simulink model "Sensor_Process"  (R2025b)
settings: Solver=VariableStepAuto  StartTime=0.0  StopTime=10.0  RelTol=1e-3
values from neighbouring files (symbols this model uses):
  sensor_distance_table = [100 80 60 40 20 5]    [run_MAIN.m]
  sensor_voltage_breakpoints = [0 1 2 3 4 5]    [run_MAIN.m]
settings Model: Creator=Mohamed  LastModifiedBy=Mohamed

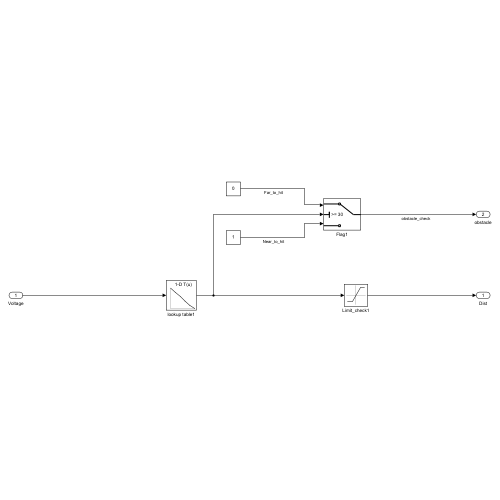
[thumbnail: Simulink's stored preview of the top-level diagram]
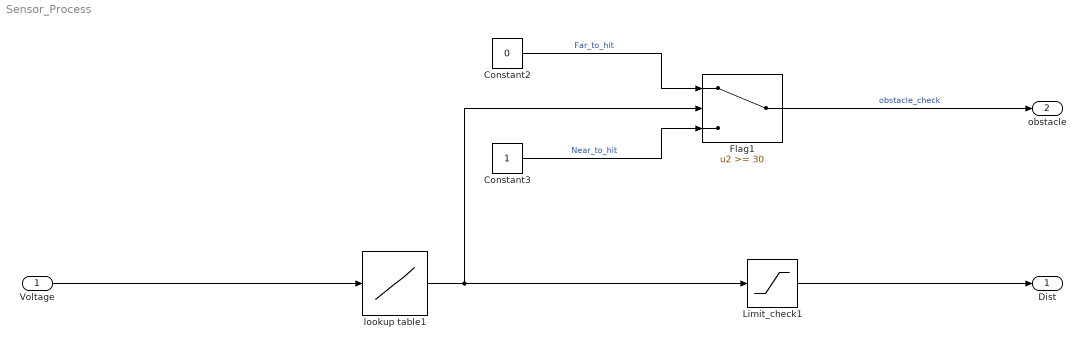
== system Sensor_Process ==
  Voltage : Inport
  Constant2 : Constant  Value=0
  Constant3 : Constant
  Flag1 : Switch  Threshold=30  OutDataTypeStr=boolean  SaturateOnIntegerOverflow=off  InputSameDT=off
  Limit_check1 : Saturate  UpperLimit=400  LowerLimit=10
  lookup table1 : Lookup_n-D  NumberOfTableDimensions=1  BreakpointsForDimension1=sensor_voltage_breakpoints  Table=sensor_distance_table  ExtrapMethod=Clip  UseLastTableValue=on  InternalRulePriority=Speed  RndMeth=Simplest
  Dist : Outport
  obstacle : Outport  Port=2
  wires:
  Limit_check1/1 -> Dist/1
  Voltage/1 -> lookup table1/1
  Constant3/1 -> Flag1/3  "Near_to_hit"
  Flag1/1 -> obstacle/1  "obstacle_check"
  Constant2/1 -> Flag1/1  "Far_to_hit"
  lookup table1/1 -> Limit_check1/1, Flag1/2
